simulink model "rate_controller"  (R2016a)
settings: Solver=VariableStepAuto  StartTime=0.0  StopTime=10.0  RelTol=1e-3
settings Model: Creator=GusBus  LastModifiedBy=GusBus
settings GRTTargetCC: GeneratePreprocessorConditionals=Use local settings

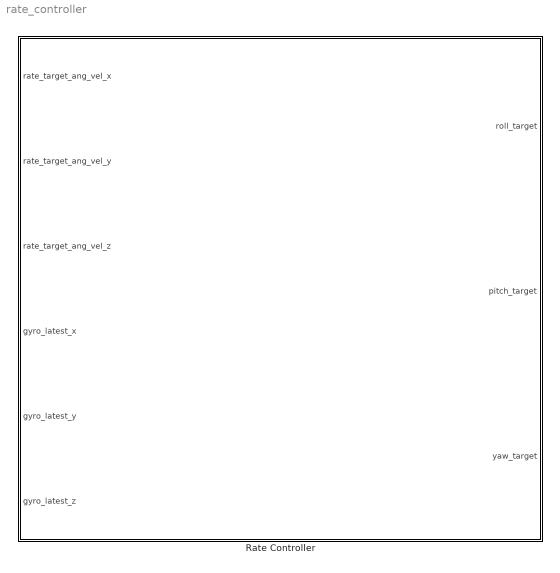
== system rate_controller ==
  Rate Controller : MATLAB Function  TreatAsAtomicUnit=on

== matlab function rate_controller/Rate Controller ==
  data: rate_target_ang_vel_x input; rate_target_ang_vel_y input; rate_target_ang_vel_z input; gyro_latest_x input; gyro_latest_y input; gyro_latest_z input; roll_target output; pitch_target output; yaw_target output
function [roll_target, pitch_target, yaw_target]  = rate_controller_run( rate_target_ang_vel_x, rate_target_ang_vel_y, rate_target_ang_vel_z , gyro_latest_x, gyro_latest_y, gyro_latest_z)
%RATE_CONTROLLER_RUN Summary of this function goes here
%   Detailed explanation goes here

update_throttle_rpy_mix();

roll_target = rate_target_to_motor_roll(gyro_latest_x, rate_target_ang_vel_x);

pitch_target = rate_target_to_motor_pitch(gyro_latest_y, rate_target_ang_vel_y);

yaw_target = rate_target_to_motor_yaw(gyro_latest_z, rate_target_ang_vel_z);

end
